simulink model "positionWalking_legacy"  (Simulink 8.3)
settings: Solver=FixedStepDiscrete  StartTime=0.0  StopTime=Config.t_end  FixedStep=Config.t_step  RelTol=1e-3
InitFcn:
  | cd(fileparts(which(bdroot)));
  | initTorqueWalking;
undefined symbols (not defined in the file): Config, DiscIntNeverNeededParam, gains, ROBOT_DOF
libraries: WBToolboxLibrary x88
(part 2 of 3)

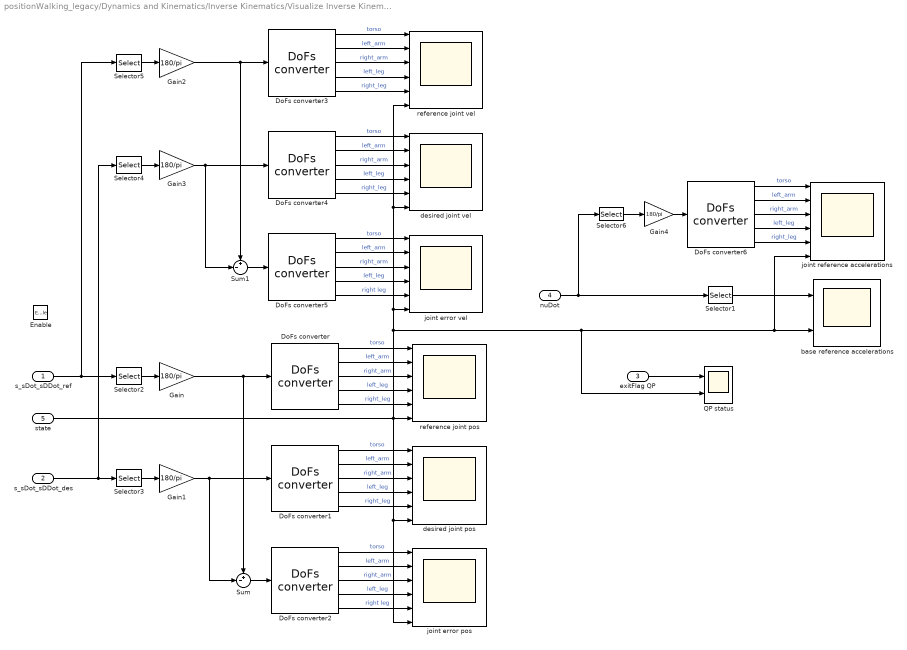
== system positionWalking_legacy/Dynamics and Kinematics/Inverse Kinematics/Visualize Inverse Kinematics ==
  s_sDot_sDDot_ref : Inport
  s_sDot_sDDot_des : Inport  Port=2
  exitFlag QP : Inport  Port=3
  nuDot : Inport  Port=4
  state : Inport  Port=5
  Enable : EnablePort
  DoFs converter{,1..6} (7 alike) : WBToolboxLibrary/Utilities/DoFs converter  yarp2WBIOption=From WBI to YARP  robotName=WBT_robotName  localName=WBT_modelName  wbiFile=WBT_wbiFilename  wbiList=WBT_wbiList
  Gain{,1..4} (5 alike) : Gain  Gain=180/pi
  QP status : Scope  NumInputPorts=2
      settings: TimeRange=auto  MaxDataPoints=5000  SaveName=ikin_QPStatus_DATA  YMin=-1.00000~0.9  YMax=1.00000~1.1  SampleTime=-1
  Selector1 : Selector  InputPortWidth=ROBOT_DOF+6  IndexOptions=Index vector (dialog)  Indices=[1:6]  OutputSizes=1
  Selector2 : Selector  NumberOfDimensions=2  InputPortWidth=ROBOT_DOF  IndexOptions=Index vector (dialog),Index vector (dialog)  Indices=[1:ROBOT_DOF],1  OutputSizes=1,1
  Selector3 : Selector  NumberOfDimensions=2  InputPortWidth=ROBOT_DOF  IndexOptions=Index vector (dialog),Index vector (dialog)  Indices=[1:ROBOT_DOF],1  OutputSizes=1,1
  Selector4 : Selector  NumberOfDimensions=2  InputPortWidth=ROBOT_DOF  IndexOptions=Index vector (dialog),Index vector (dialog)  Indices=[1:ROBOT_DOF],2  OutputSizes=1,1
  Selector5 : Selector  NumberOfDimensions=2  InputPortWidth=ROBOT_DOF  IndexOptions=Index vector (dialog),Index vector (dialog)  Indices=[1:ROBOT_DOF],2  OutputSizes=1,1
  Selector6 : Selector  InputPortWidth=ROBOT_DOF+6  IndexOptions=Index vector (dialog)  Indices=[7:ROBOT_DOF+6]  OutputSizes=1
  Sum : Sum  Inputs=+-|
  Sum1 : Sum  Inputs=+-|
  base reference accelerations : Scope  NumInputPorts=2
      settings: TimeRange=auto  MaxDataPoints=5000  SaveName=ikin_baseAcc_DATA  YMin=-0.01102~0.9  YMax=0.00514~1.1  SampleTime=-1
  desired joint pos : Scope  NumInputPorts=6
      settings: TimeRange=auto  ShowLegends=on  MaxDataPoints=5000  SaveName=ikin_s_des_DATA  YMin=-0.00195~-39.1214~-39.1221~-0.14128~-0.12031~0.9  YMax=0.02043~54.3146~54.31552~0.12783~0.13205~1.1  SampleTime=-1
  desired joint vel : Scope  NumInputPorts=6
      settings: TimeRange=auto  MaxDataPoints=5000  SaveName=ikin_sDot_des_DATA  YMin=-1.00000~-1.00000~-1.00000~-1.00000~-1.00000~0.9  YMax=1.00000~1.00000~1.00000~1.00000~1.00000~1.1  SampleTime=-1
  joint error pos : Scope  NumInputPorts=6
      settings: TimeRange=auto  MaxDataPoints=5000  SaveName=ikin_s_err_DATA  YMin=-5.9022~-0.98644~-1.02648~-5.57984~-5.5405~0.9  YMax=6.12835~0.97735~0.94334~5.54057~5.57971~1.1  SampleTime=-1
  joint error vel : Scope  NumInputPorts=6
      settings: TimeRange=auto  MaxDataPoints=5000  SaveName=ikin_sDot_err_DATA  YMin=-0.00011~-0.000021~-0.00064~-0.00028~-0.00066~0.9  YMax=0.00008~0.000046~0.00101~0.00072~0.00021~1.1  SampleTime=-1
  joint reference accelerations : Scope  NumInputPorts=6
      settings: TimeRange=auto  MaxDataPoints=5000  SaveName=ikin_sDDot_ref_DATA  YMin=-2.86444~-1.31048~-1.31054~-1.0443~-1.04238~0.9  YMax=1.2637~1.01756~1.0173~0.54022~0.54065~1.1  SampleTime=-1
  reference joint pos : Scope  NumInputPorts=6
      settings: TimeRange=auto  MaxDataPoints=5000  SaveName=ikin_s_ref_DATA  YMin=-1.73238~-39.09396~-39.16347~-0.13035~-0.1588~0.9  YMax=-0.13168~54.24597~54.26229~0.09217~0.03558~1.1  SampleTime=-1
  reference joint vel : Scope  NumInputPorts=6
      settings: TimeRange=auto  MaxDataPoints=5000  SaveName=ikin_sDot_ref_DATA  YMin=-1.00000~-1.00000~-1.00000~-1.00000~-1.00000~0.9  YMax=1.00000~1.00000~1.00000~1.00000~1.00000~1.1  SampleTime=-1
  wires:
  DoFs converter1/2 -> desired joint pos/2  "left_arm"
  DoFs converter/5 -> reference joint pos/5  "right_leg"
  DoFs converter2/1 -> joint error pos/1  "torso"
  DoFs converter/4 -> reference joint pos/4  "left_leg"
  DoFs converter/2 -> reference joint pos/2  "left_arm"
  DoFs converter1/1 -> desired joint pos/1  "torso"
  DoFs converter1/4 -> desired joint pos/4  "left_leg"
  DoFs converter1/3 -> desired joint pos/3  "right_arm"
  DoFs converter/3 -> reference joint pos/3  "right_arm"
  DoFs converter2/2 -> joint error pos/2  "left_arm"
  DoFs converter/1 -> reference joint pos/1  "torso"
  DoFs converter1/5 -> desired joint pos/5  "right_leg"
  DoFs converter2/4 -> joint error pos/4  "left_leg"
  Sum/1 -> DoFs converter2/1
  DoFs converter2/3 -> joint error pos/3  "right_arm"
  Gain/1 -> Sum/1, DoFs converter/1
  Gain1/1 -> Sum/2, DoFs converter1/1
  DoFs converter4/2 -> desired joint vel/2  "left_arm"
  DoFs converter3/5 -> reference joint vel/5  "right_leg"
  DoFs converter5/1 -> joint error vel/1  "torso"
  DoFs converter3/4 -> reference joint vel/4  "left_leg"
  DoFs converter3/2 -> reference joint vel/2  "left_arm"
  s_sDot_sDDot_ref/1 -> Selector5/1, Selector2/1
  DoFs converter4/1 -> desired joint vel/1  "torso"
  DoFs converter4/4 -> desired joint vel/4  "left_leg"
  DoFs converter4/3 -> desired joint vel/3  "right_arm"
  DoFs converter3/3 -> reference joint vel/3  "right_arm"
  DoFs converter5/2 -> joint error vel/2  "left_arm"
  DoFs converter3/1 -> reference joint vel/1  "torso"
  s_sDot_sDDot_des/1 -> Selector4/1, Selector3/1
  DoFs converter4/5 -> desired joint vel/5  "right_leg"
  DoFs converter5/4 -> joint error vel/4  "left_leg"
  Sum1/1 -> DoFs converter5/1
  DoFs converter5/3 -> joint error vel/3  "right_arm"
  Gain2/1 -> Sum1/1, DoFs converter3/1
  Gain3/1 -> Sum1/2, DoFs converter4/1
  DoFs converter5/5 -> joint error vel/5  "right leg"
  DoFs converter2/5 -> joint error pos/5  "right leg"
  Selector1/1 -> base reference accelerations/1
  Selector2/1 -> Gain/1
  Selector3/1 -> Gain1/1
  Selector4/1 -> Gain3/1
  Selector5/1 -> Gain2/1
  DoFs converter6/5 -> joint reference accelerations/5  "right_leg"
  DoFs converter6/1 -> joint reference accelerations/1  "torso"
  DoFs converter6/4 -> joint reference accelerations/4  "left_leg"
  DoFs converter6/3 -> joint reference accelerations/3  "right_arm"
  DoFs converter6/2 -> joint reference accelerations/2  "left_arm"
  nuDot/1 -> Selector6/1, Selector1/1
  Gain4/1 -> DoFs converter6/1
  Selector6/1 -> Gain4/1
  state/1 -> reference joint vel/6, desired joint vel/6, joint error vel/6, QP status/2, joint reference accelerations/6, base reference accelerations/2, joint error pos/6, desired joint pos/6, reference joint pos/6
  exitFlag QP/1 -> QP status/1

== system positionWalking_legacy/Dynamics and Kinematics/Task Accelerations/ComputeTasksPoseAndVelocity ==
  J_LFoot : Inport
  J_RFoot : Inport  Port=2
  J_CoM : Inport  Port=3
  J_Rot_task : Inport  Port=4
  s : Inport  Port=5
  w_H_b : Inport  Port=6
  nu : Inport  Port=7
  Compose Task Pose and Velocity : MATLAB Function  TreatAsAtomicUnit=on
      settings: PermitHierarchicalResolution=ParametersOnly
  Product{,1..3} (4 alike) : Product  Multiplication=Matrix(*)
  Task position and orientation : Subsystem
  pos_vel_CoM : Outport
  pose_vel_LFoot : Outport  Port=2
  pose_vel_RFoot : Outport  Port=3
  orient_vel_Rot_task : Outport  Port=4
  wires:
  Compose Task Pose and Velocity/3(pose_vel_RFoot) -> pose_vel_RFoot/1
  Compose Task Pose and Velocity/2(pose_vel_LFoot) -> pose_vel_LFoot/1
  Compose Task Pose and Velocity/1(pos_vel_CoM) -> pos_vel_CoM/1
  Compose Task Pose and Velocity/4(orient_vel_Rot_task) -> orient_vel_Rot_task/1
  nu/1 -> Product1/2, Product/2, Product2/2, Product3/2
  J_Rot_task/1 -> Product3/1
  Product/1 -> Compose Task Pose and Velocity/1(vel_CoM)
  Product1/1 -> Compose Task Pose and Velocity/2(vel_LFoot)
  Product2/1 -> Compose Task Pose and Velocity/3(vel_RFoot)
  Product3/1 -> Compose Task Pose and Velocity/4(vel_Rot_task)
  s/1 -> Task position and orientation/1(s)
  w_H_b/1 -> Task position and orientation/2(w_H_b)
  Task position and orientation/1(w_H_CoM) -> Compose Task Pose and Velocity/5(w_H_CoM)
  Task position and orientation/2(w_H_l_sole) -> Compose Task Pose and Velocity/6(w_H_l_sole)
  Task position and orientation/3(w_H_r_sole) -> Compose Task Pose and Velocity/7(w_H_r_sole)
  Task position and orientation/4(w_H_Rot_task) -> Compose Task Pose and Velocity/8(w_H_Rot_task)
  J_RFoot/1 -> Product2/1
  J_LFoot/1 -> Product1/1
  J_CoM/1 -> Product/1

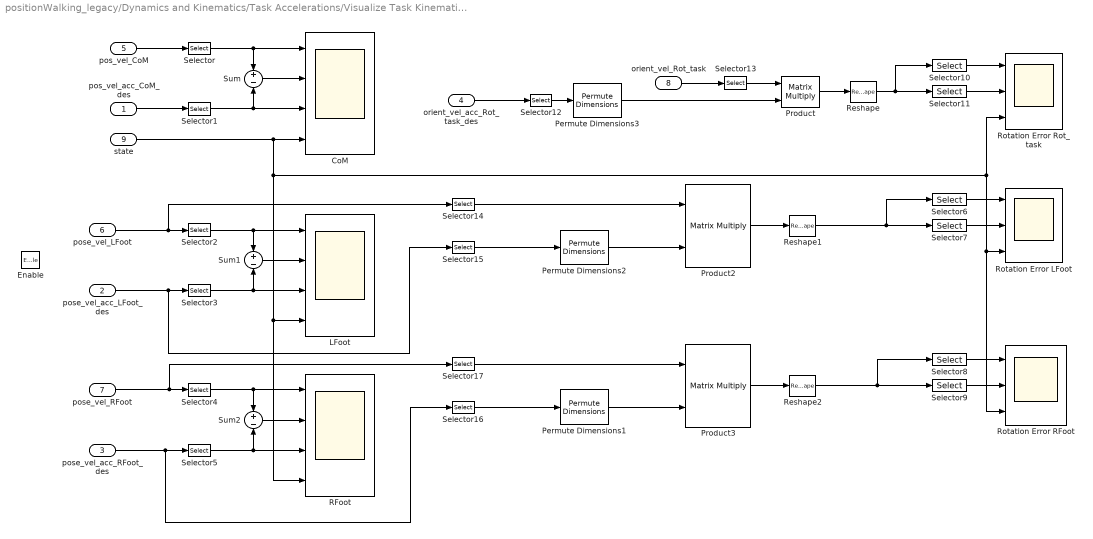
== system positionWalking_legacy/Dynamics and Kinematics/Task Accelerations/Visualize Task Kinematics ==
  pos_vel_acc_CoM_des : Inport
  pose_vel_acc_LFoot_des : Inport  Port=2
  pose_vel_acc_RFoot_des : Inport  Port=3
  orient_vel_acc_Rot_task_des : Inport  Port=4
  pos_vel_CoM : Inport  Port=5
  pose_vel_LFoot : Inport  Port=6
  pose_vel_RFoot : Inport  Port=7
  orient_vel_Rot_task : Inport  Port=8
  state : Inport  Port=9
  Enable : EnablePort
  CoM : Scope  NumInputPorts=4
      settings: TimeRange=auto  MaxDataPoints=5000  SaveName=forKin_CoM_DATA  YMin=-0.16396~-0.00327~-0.16319~0.9  YMax=0.58824~0.00906~0.58815~1.1  SampleTime=-1
  LFoot : Scope  NumInputPorts=4
      settings: TimeRange=auto  MaxDataPoints=5000  SaveName=forKin_LFoot_DATA  YMin=-0.00000000000000042~-0.00000000000000042~-0.000000000000000002~0.9  YMax=0.00000000000000045~0.00000000000000045~0.000000000000000017~1.1  SampleTime=-1
  Permute Dimensions1 : PermuteDimensions
  Permute Dimensions2 : PermuteDimensions
  Permute Dimensions3 : PermuteDimensions
  Product : Product  Multiplication=Matrix(*)
  Product2 : Product  Multiplication=Matrix(*)
  Product3 : Product  Multiplication=Matrix(*)
  RFoot : Scope  NumInputPorts=4
      settings: TimeRange=auto  MaxDataPoints=5000  SaveName=forKin_RFoot_DATA  YMin=-0.15347~-0.00033~-0.15317~0.9  YMax=0.01708~0.00035~0.01701~1.1  SampleTime=-1
  Reshape : Reshape
  Reshape1 : Reshape
  Reshape2 : Reshape
  Rotation Error LFoot : Scope  NumInputPorts=3
      settings: TimeRange=auto  MaxDataPoints=5000  SaveName=rotErr_LFoot_DATA  YMin=0.9999999999999994~-0.00000000000000006~0.9  YMax=1.0000000000000009~0.00000000000000006~1.1  SampleTime=-1
  Rotation Error RFoot : Scope  NumInputPorts=3
      settings: TimeRange=auto  MaxDataPoints=5000  SaveName=rotErr_RFoot_DATA  YMin=0.99999975~-0.00082~0.9  YMax=1.00000003~0.00082~1.1  SampleTime=-1
  Rotation Error Rot_task : Scope  NumInputPorts=3
      settings: TimeRange=auto  MaxDataPoints=5000  SaveName=rotErr_Root_DATA  YMin=0.99623~-0.1023~0.9  YMax=1.00042~0.1023~1.1  SampleTime=-1
  Selector{,1..5} (6 alike) : Selector  NumberOfDimensions=2  InputPortWidth=3  IndexOptions=Index vector (dialog),Index vector (dialog)  Indices=[1:3],1  OutputSizes=1,1
  Selector10 : Selector  InputPortWidth=9  IndexOptions=Index vector (dialog)  Indices=[1 5 9]  OutputSizes=1
  Selector11 : Selector  InputPortWidth=9  IndexOptions=Index vector (dialog)  Indices=[2 3 4 6 7 8]  OutputSizes=1
  Selector12 : Selector  NumberOfDimensions=2  InputPortWidth=3  IndexOptions=Index vector (dialog),Index vector (dialog)  Indices=[1:3],[1:3]  OutputSizes=1,1
  Selector13 : Selector  NumberOfDimensions=2  InputPortWidth=3  IndexOptions=Index vector (dialog),Index vector (dialog)  Indices=[1:3],[1:3]  OutputSizes=1,1
  Selector{14..17} (4 alike) : Selector  NumberOfDimensions=2  InputPortWidth=3  IndexOptions=Index vector (dialog),Index vector (dialog)  Indices=[4:6],[1:3]  OutputSizes=1,1
  Selector6 : Selector  InputPortWidth=9  IndexOptions=Index vector (dialog)  Indices=[1 5 9]  OutputSizes=1
  Selector7 : Selector  InputPortWidth=9  IndexOptions=Index vector (dialog)  Indices=[2 3 4 6 7 8]  OutputSizes=1
  Selector8 : Selector  InputPortWidth=9  IndexOptions=Index vector (dialog)  Indices=[1 5 9]  OutputSizes=1
  Selector9 : Selector  InputPortWidth=9  IndexOptions=Index vector (dialog)  Indices=[2 3 4 6 7 8]  OutputSizes=1
  Sum : Sum  Inputs=+|-
  Sum1 : Sum  Inputs=+|-
  Sum2 : Sum  Inputs=+|-
  wires:
  Selector/1 -> Sum/1, CoM/1
  Selector1/1 -> CoM/3, Sum/2
  Sum/1 -> CoM/2
  pos_vel_CoM/1 -> Selector/1
  pos_vel_acc_CoM_des/1 -> Selector1/1
  Selector2/1 -> LFoot/1, Sum1/1
  Selector3/1 -> LFoot/3, Sum1/2
  Sum1/1 -> LFoot/2
  Selector4/1 -> RFoot/1, Sum2/1
  Selector5/1 -> RFoot/3, Sum2/2
  Sum2/1 -> RFoot/2
  pose_vel_RFoot/1 -> Selector17/1, Selector4/1
  state/1 -> RFoot/4, LFoot/4, Rotation Error RFoot/3, Rotation Error LFoot/3, Rotation Error Rot_task/3, CoM/4
  pose_vel_acc_RFoot_des/1 -> Selector5/1, Selector16/1
  Permute Dimensions2/1 -> Product2/2
  Permute Dimensions1/1 -> Product3/2
  Permute Dimensions3/1 -> Product/2
  Product2/1 -> Reshape1/1
  Product3/1 -> Reshape2/1
  Product/1 -> Reshape/1
  Selector13/1 -> Product/1
  pose_vel_LFoot/1 -> Selector14/1, Selector2/1
  Reshape1/1 -> Selector6/1, Selector7/1
  Reshape2/1 -> Selector8/1, Selector9/1
  Reshape/1 -> Selector10/1, Selector11/1
  Selector7/1 -> Rotation Error LFoot/2
  Selector6/1 -> Rotation Error LFoot/1
  Selector8/1 -> Rotation Error RFoot/1
  Selector9/1 -> Rotation Error RFoot/2
  Selector10/1 -> Rotation Error Rot_task/1
  Selector11/1 -> Rotation Error Rot_task/2
  Selector12/1 -> Permute Dimensions3/1
  pose_vel_acc_LFoot_des/1 -> Selector15/1, Selector3/1
  orient_vel_acc_Rot_task_des/1 -> Selector12/1
  orient_vel_Rot_task/1 -> Selector13/1
  Selector14/1 -> Product2/1
  Selector15/1 -> Permute Dimensions2/1
  Selector16/1 -> Permute Dimensions1/1
  Selector17/1 -> Product3/1

== system positionWalking_legacy/Robot State and References/Reference Velocities and Accelerations/Reference Orientations ==
  w_R_LFoot_des : Inport
  w_R_RFoot_des : Inport  Port=2
  w_R_Rot_task_des : Inport  Port=3
  Compute Reference Angular Accelerations : MATLAB Function  TreatAsAtomicUnit=on
      settings: PermitHierarchicalResolution=ParametersOnly
  Compute Rotation Matrix Derivative : MATLAB Function  TreatAsAtomicUnit=on
      settings: PermitHierarchicalResolution=ParametersOnly
  Discrete-Time Integrator : DiscreteIntegrator  InitialCondition=zeros(3,1)  InitialConditionSetting=State (most efficient)  SampleTime=Config.t_step  ICPrevOutput=DiscIntNeverNeededParam  ICPrevScaledInput=DiscIntNeverNeededParam
  Discrete-Time Integrator1 : DiscreteIntegrator  InitialConditionSource=external  InitialCondition=zeros(3,1)  InitialConditionSetting=State (most efficient)  SampleTime=Config.t_step  ICPrevOutput=DiscIntNeverNeededParam  ICPrevScaledInput=DiscIntNeverNeededParam
  Discrete-Time Integrator2 : DiscreteIntegrator  InitialConditionSource=external  InitialCondition=zeros(3,1)  InitialConditionSetting=State (most efficient)  SampleTime=Config.t_step  ICPrevOutput=DiscIntNeverNeededParam  ICPrevScaledInput=DiscIntNeverNeededParam
  Discrete-Time Integrator3 : DiscreteIntegrator  InitialCondition=zeros(3,1)  InitialConditionSetting=State (most efficient)  SampleTime=Config.t_step  ICPrevOutput=DiscIntNeverNeededParam  ICPrevScaledInput=DiscIntNeverNeededParam
  Discrete-Time Integrator4 : DiscreteIntegrator  InitialCondition=zeros(3,1)  InitialConditionSetting=State (most efficient)  SampleTime=Config.t_step  ICPrevOutput=DiscIntNeverNeededParam  ICPrevScaledInput=DiscIntNeverNeededParam
  Discrete-Time Integrator5 : DiscreteIntegrator  InitialConditionSource=external  InitialCondition=zeros(3,1)  InitialConditionSetting=State (most efficient)  SampleTime=Config.t_step  ICPrevOutput=DiscIntNeverNeededParam  ICPrevScaledInput=DiscIntNeverNeededParam
  Matrix Concatenate5 : Concatenate  NumInputs=3  Mode=Multidimensional array  ConcatenateDimension=2
  Matrix Concatenate6 : Concatenate  NumInputs=3  Mode=Multidimensional array  ConcatenateDimension=2
  Matrix Concatenate7 : Concatenate  NumInputs=3  Mode=Multidimensional array  ConcatenateDimension=2
  Visualize Desired Rotations : Subsystem
  "holder " : WBToolboxLibrary/Utilities/holder 
  holder 1 : WBToolboxLibrary/Utilities/holder 
  holder 2 : WBToolboxLibrary/Utilities/holder 
  orient_vel_acc_LFoot_des : Outport
  orient_vel_acc_RFoot_des : Outport  Port=2
  orient_vel_acc_Rot_task_des : Outport  Port=3
  wires:
  Compute Reference Angular Accelerations/1(omegaDot_LFoot) -> Discrete-Time Integrator/1, Matrix Concatenate6/3, Visualize Desired Rotations/4(omegaDot_LFoot)
  Compute Reference Angular Accelerations/3(omegaDot_Rot_task) -> Discrete-Time Integrator4/1, Matrix Concatenate7/3, Visualize Desired Rotations/6(omegaDot_Root)
  Discrete-Time Integrator/1 -> Compute Rotation Matrix Derivative/1(omega_LFoot), Matrix Concatenate6/2, Compute Reference Angular Accelerations/7(omega_LFoot), Visualize Desired Rotations/9(omega_LFoot)
  Discrete-Time Integrator3/1 -> Compute Rotation Matrix Derivative/2(omega_RFoot), Matrix Concatenate5/2, Compute Reference Angular Accelerations/8(omega_RFoot), Visualize Desired Rotations/8(omega_RFoot)
  Discrete-Time Integrator4/1 -> Compute Rotation Matrix Derivative/3(omega_Rot_task), Matrix Concatenate7/2, Compute Reference Angular Accelerations/9(omega_Rot_task), Visualize Desired Rotations/7(omega_Rot_task)
  Compute Rotation Matrix Derivative/1(RDot_LFoot) -> Discrete-Time Integrator2/1
  Compute Rotation Matrix Derivative/2(RDot_RFoot) -> Discrete-Time Integrator5/1
  Compute Rotation Matrix Derivative/3(RDot_Rot_task) -> Discrete-Time Integrator1/1
  Discrete-Time Integrator2/1 -> Compute Rotation Matrix Derivative/4(w_R_LFoot), Matrix Concatenate6/1, Visualize Desired Rotations/10(w_R_LFoot), Compute Reference Angular Accelerations/4(w_R_LFoot)
  Discrete-Time Integrator5/1 -> Compute Rotation Matrix Derivative/5(w_R_RFoot), Compute Reference Angular Accelerations/5(w_R_RFoot), Visualize Desired Rotations/11(w_R_RFoot), Matrix Concatenate5/1
  Discrete-Time Integrator1/1 -> Compute Rotation Matrix Derivative/6(w_R_Rot_task), Compute Reference Angular Accelerations/6(w_R_Rot_task), Matrix Concatenate7/1, Visualize Desired Rotations/12(w_R_Rot_task)
  "holder "/1 -> Discrete-Time Integrator2/2
  holder 2/1 -> Discrete-Time Integrator5/2
  holder 1/1 -> Discrete-Time Integrator1/2
  Compute Reference Angular Accelerations/2(omegaDot_RFoot) -> Discrete-Time Integrator3/1, Matrix Concatenate5/3, Visualize Desired Rotations/5(omegaDot_RFoot)
  Matrix Concatenate6/1 -> orient_vel_acc_LFoot_des/1
  Matrix Concatenate5/1 -> orient_vel_acc_RFoot_des/1
  Matrix Concatenate7/1 -> orient_vel_acc_Rot_task_des/1
  w_R_LFoot_des/1 -> Visualize Desired Rotations/1(w_R_LFoot_des), "holder "/1, Compute Reference Angular Accelerations/1(w_R_LFoot_des)
  w_R_RFoot_des/1 -> Compute Reference Angular Accelerations/2(w_R_RFoot_des), Visualize Desired Rotations/2(w_R_RFoot_des), holder 2/1
  w_R_Rot_task_des/1 -> Compute Reference Angular Accelerations/3(w_R_Rot_task_des), Visualize Desired Rotations/3(w_R_Rot_task_des), holder 1/1

== system positionWalking_legacy/Robot State and References/Reference Velocities and Accelerations/Reference Positions ==
  pos_CoM_des : Inport
  pos_LFoot_des : Inport  Port=2
  pos_RFoot_des : Inport  Port=3
  s_des : Inport  Port=4
  Matrix Concatenate1 : Concatenate  NumInputs=3  Mode=Multidimensional array  ConcatenateDimension=2
  Matrix Concatenate2 : Concatenate  NumInputs=4  Mode=Multidimensional array  ConcatenateDimension=2
  Matrix Concatenate3 : Concatenate  NumInputs=4  Mode=Multidimensional array  ConcatenateDimension=2
  Matrix Concatenate4 : Concatenate  NumInputs=3  Mode=Multidimensional array  ConcatenateDimension=2
  Minimum Jerk Trajectory Generator{,1..3} (4 alike) : WBToolboxLibrary/Utilities/Minimum Jerk Trajectory Generator  externalSettlingTime=on  settlingTime=3  sampleTime=Config.t_step  resetOnSettlingTime=off  firstDerivatives=on  secondDerivatives=on  explicitInitialValue=off
  Settling time1 : Constant  Value=zeros(3,2)
  gains smoothing time : Constant  Value=Config.t_smoothingTimeRef
  pos_vel_acc_CoM_des : Outport
  s_sDot_sDDot_ref : Outport  Port=2
  pos_vel_acc_LFoot_des : Outport  Port=3
  pos_vel_acc_RFoot_des : Outport  Port=4
  wires:
  Minimum Jerk Trajectory Generator2/2 -> Matrix Concatenate3/2
  pos_LFoot_des/1 -> Minimum Jerk Trajectory Generator2/1
  pos_RFoot_des/1 -> Minimum Jerk Trajectory Generator3/1
  Minimum Jerk Trajectory Generator2/3 -> Matrix Concatenate3/3
  Minimum Jerk Trajectory Generator2/1 -> Matrix Concatenate3/1
  Minimum Jerk Trajectory Generator1/3 -> Matrix Concatenate1/3
  Matrix Concatenate1/1 -> s_sDot_sDDot_ref/1
  Matrix Concatenate4/1 -> pos_vel_acc_CoM_des/1
  Minimum Jerk Trajectory Generator1/1 -> Matrix Concatenate1/1
  pos_CoM_des/1 -> Minimum Jerk Trajectory Generator/1
  Minimum Jerk Trajectory Generator/3 -> Matrix Concatenate4/3
  Minimum Jerk Trajectory Generator/2 -> Matrix Concatenate4/2
  Minimum Jerk Trajectory Generator1/2 -> Matrix Concatenate1/2
  Minimum Jerk Trajectory Generator3/3 -> Matrix Concatenate2/3
  Matrix Concatenate3/1 -> pos_vel_acc_LFoot_des/1
  Matrix Concatenate2/1 -> pos_vel_acc_RFoot_des/1
  Minimum Jerk Trajectory Generator/1 -> Matrix Concatenate4/1
  Minimum Jerk Trajectory Generator3/2 -> Matrix Concatenate2/2
  s_des/1 -> Minimum Jerk Trajectory Generator1/1
  Settling time1/1 -> Matrix Concatenate2/4, Matrix Concatenate3/4
  gains smoothing time/1 -> Minimum Jerk Trajectory Generator/2, Minimum Jerk Trajectory Generator1/2, Minimum Jerk Trajectory Generator2/2, Minimum Jerk Trajectory Generator3/2
  Minimum Jerk Trajectory Generator3/1 -> Matrix Concatenate2/1

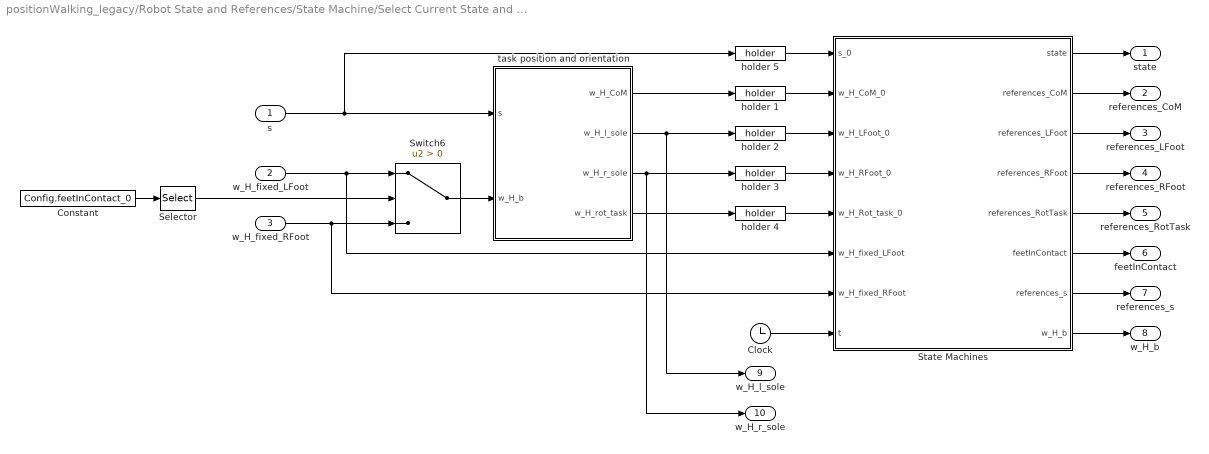
== system positionWalking_legacy/Robot State and References/State Machine/Select Current State and References ==
  s : Inport
  w_H_fixed_LFoot : Inport  Port=2
  w_H_fixed_RFoot : Inport  Port=3
  Clock : Clock
  Constant : Constant  Value=Config.feetInContact_0
  Selector : Selector  InputPortWidth=2  IndexOptions=Index vector (dialog)  Indices=1  OutputSizes=1
  State Machines : MATLAB Function  TreatAsAtomicUnit=on
      settings: PermitHierarchicalResolution=ParametersOnly
  Switch6 : Switch  Criteria=u2 > Threshold
  holder {1..5} (5 alike) : WBToolboxLibrary/Utilities/holder 
  task position and orientation : Subsystem
  state : Outport
  references_CoM : Outport  Port=2
  references_LFoot : Outport  Port=3
  references_RFoot : Outport  Port=4
  references_RotTask : Outport  Port=5
  feetInContact : Outport  Port=6
  references_s : Outport  Port=7
  w_H_b : Outport  Port=8
  w_H_l_sole : Outport  Port=9
  w_H_r_sole : Outport  Port=10
  wires:
  Switch6/1 -> task position and orientation/2(w_H_b)
  w_H_fixed_LFoot/1 -> Switch6/1, State Machines/6(w_H_fixed_LFoot)
  Constant/1 -> Selector/1
  State Machines/3(references_LFoot) -> references_LFoot/1
  task position and orientation/2(w_H_l_sole) -> holder 2/1, w_H_l_sole/1
  holder 3/1 -> State Machines/4(w_H_RFoot_0)
  State Machines/5(references_RotTask) -> references_RotTask/1
  State Machines/4(references_RFoot) -> references_RFoot/1
  s/1 -> task position and orientation/1(s), holder 5/1
  holder 4/1 -> State Machines/5(w_H_Rot_task_0)
  task position and orientation/1(w_H_CoM) -> holder 1/1
  holder 2/1 -> State Machines/3(w_H_LFoot_0)
  task position and orientation/4(w_H_rot_task) -> holder 4/1
  Selector/1 -> Switch6/2
  State Machines/1(state) -> state/1
  w_H_fixed_RFoot/1 -> State Machines/7(w_H_fixed_RFoot), Switch6/3
  State Machines/6(feetInContact) -> feetInContact/1
  task position and orientation/3(w_H_r_sole) -> holder 3/1, w_H_r_sole/1
  Clock/1 -> State Machines/8(t)
  State Machines/7(references_s) -> references_s/1
  State Machines/2(references_CoM) -> references_CoM/1
  State Machines/8(w_H_b) -> w_H_b/1
  holder 1/1 -> State Machines/2(w_H_CoM_0)
  holder 5/1 -> State Machines/1(s_0)

== system positionWalking_legacy/Robot State and References/State Machine/World to fixed link transform ==
  s : Inport
  w_H_b : Inport  Port=2
  IMU port : Inport  Port=3
  left foot : WBToolboxLibrary/wholeBodyModel/Kinematics/Forward Kinematics  frameName=Frames.LEFT_FOOT  robotName=WBT_robotName  localName=WBT_modelName  wbiFile=WBT_wbiFilename  wbiList=WBT_wbiList
  right foot : WBToolboxLibrary/wholeBodyModel/Kinematics/Forward Kinematics  frameName=Frames.RIGHT_FOOT  robotName=WBT_robotName  localName=WBT_modelName  wbiFile=WBT_wbiFilename  wbiList=WBT_wbiList
  w_H_b with left foot fixed : Subsystem
  w_H_b with right foot fixed : Subsystem
  w_H_fixed_LFoot : Outport
  w_H_fixed_RFoot : Outport  Port=2
  wires:
  s/1 -> right foot/2, w_H_b with right foot fixed/1(s), w_H_b with left foot fixed/1(s), left foot/2
  w_H_b/1 -> left foot/1, right foot/1
  w_H_b with right foot fixed/1(w_H_b) -> w_H_fixed_RFoot/1
  IMU port/1 -> w_H_b with left foot fixed/2(inertial), w_H_b with right foot fixed/2(inertial)
  right foot/1 -> w_H_b with right foot fixed/3(w_H_fixedLink)
  w_H_b with left foot fixed/1(w_H_b) -> w_H_fixed_LFoot/1
  left foot/1 -> w_H_b with left foot fixed/3(w_H_fixedLink)

== system positionWalking_legacy/Robot State and References/State Machine/compute state velocity ==
  s : Inport
  w_H_b : Inport  Port=2
  "feetInContact " : Inport  Port=3
  Compute Base Velocity : MATLAB Function  TreatAsAtomicUnit=on
      settings: PermitHierarchicalResolution=ParametersOnly
  Feet Jacobians : Subsystem
  Get Estimate : WBToolboxLibrary/wholeBodyStates/Get Estimate  estimateType=Joints Velocity  robotName=WBT_robotName  localName=WBT_modelName  wbiFile=WBT_wbiFilename  wbiList=WBT_wbiList
  Mux : Mux  Inputs=2
  nu : Outport
  wires:
  Get Estimate/1 -> Mux/2, Compute Base Velocity/4(sDot)
  Mux/1 -> nu/1
  "feetInContact "/1 -> Compute Base Velocity/3(feetInContact)
  Compute Base Velocity/1(nu_b) -> Mux/1
  s/1 -> Feet Jacobians/1(s)
  w_H_b/1 -> Feet Jacobians/2(w_H_b)
  Feet Jacobians/1(J_LFoot) -> Compute Base Velocity/1(J_LeftFoot)
  Feet Jacobians/2(J_RFoot) -> Compute Base Velocity/2(J_RightFoot)

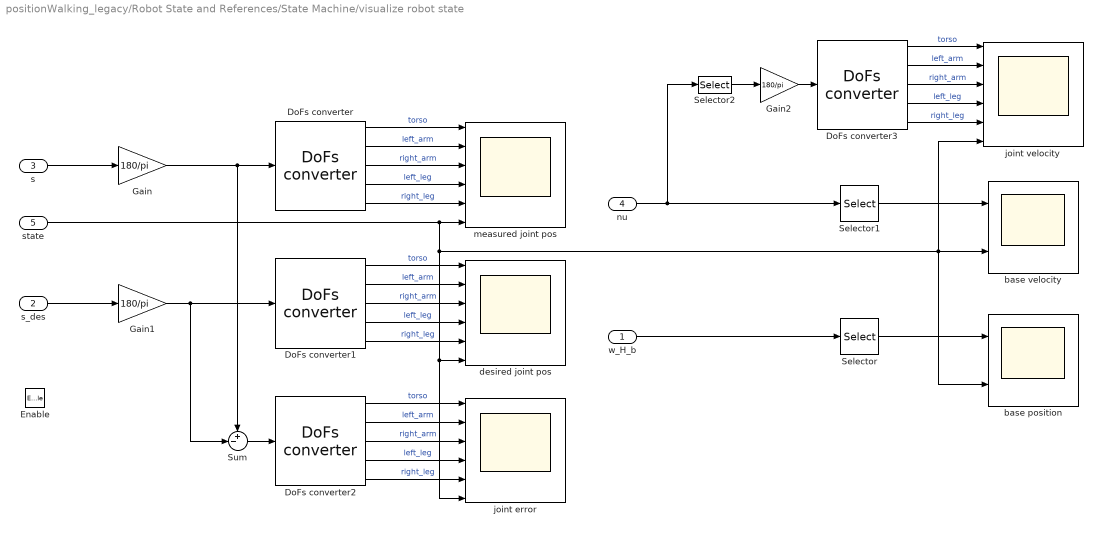
== system positionWalking_legacy/Robot State and References/State Machine/visualize robot state ==
  w_H_b : Inport
  s_des : Inport  Port=2
  s : Inport  Port=3
  nu : Inport  Port=4
  state : Inport  Port=5
  Enable : EnablePort
  DoFs converter{,1..3} (4 alike) : WBToolboxLibrary/Utilities/DoFs converter  yarp2WBIOption=From WBI to YARP  robotName=WBT_robotName  localName=WBT_modelName  wbiFile=WBT_wbiFilename  wbiList=WBT_wbiList
  Gain : Gain  Gain=180/pi
  Gain1 : Gain  Gain=180/pi
  Gain2 : Gain  Gain=180/pi
  Selector : Selector  NumberOfDimensions=2  InputPortWidth=3  IndexOptions=Index vector (dialog),Index vector (dialog)  Indices=[1:3],4  OutputSizes=1,1
  Selector1 : Selector  InputPortWidth=ROBOT_DOF+6  IndexOptions=Index vector (dialog)  Indices=[1:6]  OutputSizes=1
  Selector2 : Selector  InputPortWidth=ROBOT_DOF+6  IndexOptions=Index vector (dialog)  Indices=[7:ROBOT_DOF+6]  OutputSizes=1
  Sum : Sum  Inputs=+-|
  base position : Scope  NumInputPorts=2
      settings: TimeRange=auto  MaxDataPoints=5000  SaveName=basePos_DATA  YMin=-0.15075~0.9  YMax=0.68063~1.1  SampleTime=-1
  base velocity : Scope  NumInputPorts=2
      settings: TimeRange=auto  MaxDataPoints=5000  SaveName=baseVel_DATA  YMin=-0.00012~0.9  YMax=0.00016~1.1  SampleTime=-1
  desired joint pos : Scope  NumInputPorts=6
      settings: TimeRange=auto  MaxDataPoints=5000  SaveName=jointDes_DATA  YMin=-1.73238~-39.09396~-39.16347~-0.13035~-0.1588~0.9  YMax=-0.13168~54.24597~54.26229~0.09217~0.03558~1.1  SampleTime=-1
  joint error : Scope  NumInputPorts=6
      settings: TimeRange=auto  MaxDataPoints=5000  SaveName=jointErr_DATA  YMin=-0.10928~-0.03665~-0.06329~-0.00446~-0.00535~0.9  YMax=0.98348~0.04341~0.18869~0.01039~0.01469~1.1  SampleTime=-1
  joint velocity : Scope  NumInputPorts=6
      settings: TimeRange=auto  MaxDataPoints=5000  SaveName=jointVel_DATA  YMin=-0.03366~-0.02028~-0.03366~-0.01001~-0.00754~0.9  YMax=0.16882~0.03011~0.03479~0.00711~0.00828~1.1  SampleTime=-1
  measured joint pos : Scope  NumInputPorts=6
      settings: TimeRange=auto  MaxDataPoints=5000  SaveName=jointPos_DATA  YMin=-1.7483~-39.13033~-39.17068~-0.13107~-0.16256~0.9  YMax=0.01165~54.28691~54.29724~0.09225~0.036~1.1  SampleTime=-1
  wires:
  DoFs converter1/2 -> desired joint pos/2  "left_arm"
  DoFs converter/5 -> measured joint pos/5  "right_leg"
  DoFs converter2/1 -> joint error/1  "torso"
  DoFs converter/4 -> measured joint pos/4  "left_leg"
  DoFs converter/2 -> measured joint pos/2  "left_arm"
  s/1 -> Gain/1
  DoFs converter1/1 -> desired joint pos/1  "torso"
  DoFs converter1/4 -> desired joint pos/4  "left_leg"
  DoFs converter1/3 -> desired joint pos/3  "right_arm"
  DoFs converter/3 -> measured joint pos/3  "right_arm"
  DoFs converter2/5 -> joint error/5  "right_leg"
  DoFs converter2/2 -> joint error/2  "left_arm"
  DoFs converter/1 -> measured joint pos/1  "torso"
  s_des/1 -> Gain1/1
  DoFs converter1/5 -> desired joint pos/5  "right_leg"
  DoFs converter2/4 -> joint error/4  "left_leg"
  Sum/1 -> DoFs converter2/1
  DoFs converter2/3 -> joint error/3  "right_arm"
  DoFs converter3/5 -> joint velocity/5  "right_leg"
  DoFs converter3/1 -> joint velocity/1  "torso"
  DoFs converter3/4 -> joint velocity/4  "left_leg"
  DoFs converter3/3 -> joint velocity/3  "right_arm"
  DoFs converter3/2 -> joint velocity/2  "left_arm"
  nu/1 -> Selector2/1, Selector1/1
  w_H_b/1 -> Selector/1
  Gain/1 -> Sum/1, DoFs converter/1
  Gain1/1 -> Sum/2, DoFs converter1/1
  Gain2/1 -> DoFs converter3/1
  Selector/1 -> base position/1
  Selector2/1 -> Gain2/1
  state/1 -> measured joint pos/6, joint velocity/6, base velocity/2, base position/2, joint error/6, desired joint pos/6
  Selector1/1 -> base velocity/1

== system positionWalking_legacy/Dynamics and Kinematics/Initial Conditions/compute state velocity/Feet Jacobians ==
  s : Inport
  w_H_b : Inport  Port=2
  Jacobian LFoot : WBToolboxLibrary/wholeBodyModel/Jacobians/Jacobian  frameName=Frames.LEFT_FOOT  robotName=WBT_robotName  localName=WBT_modelName  wbiFile=WBT_wbiFilename  wbiList=WBT_wbiList
  Jacobian RFoot : WBToolboxLibrary/wholeBodyModel/Jacobians/Jacobian  frameName=Frames.RIGHT_FOOT  robotName=WBT_robotName  localName=WBT_modelName  wbiFile=WBT_wbiFilename  wbiList=WBT_wbiList
  J_LFoot : Outport
  J_RFoot : Outport  Port=2
  wires:
  Jacobian LFoot/1 -> J_LFoot/1
  Jacobian RFoot/1 -> J_RFoot/1
  w_H_b/1 -> Jacobian RFoot/1, Jacobian LFoot/1
  s/1 -> Jacobian LFoot/2, Jacobian RFoot/2

== system positionWalking_legacy/Dynamics and Kinematics/Inverse Kinematics/ComputeTasksPoseAndVelocity/Task position and orientation ==
  s : Inport
  w_H_b : Inport  Port=2
  CoM : WBToolboxLibrary/wholeBodyModel/Kinematics/Forward Kinematics  frameName=Frames.COM  robotName=WBT_robotName  localName=WBT_modelName  wbiFile=WBT_wbiFilename  wbiList=WBT_wbiList
  LFoot : WBToolboxLibrary/wholeBodyModel/Kinematics/Forward Kinematics  frameName=Frames.LEFT_FOOT  robotName=WBT_robotName  localName=WBT_modelName  wbiFile=WBT_wbiFilename  wbiList=WBT_wbiList
  RFoot : WBToolboxLibrary/wholeBodyModel/Kinematics/Forward Kinematics  frameName=Frames.RIGHT_FOOT  robotName=WBT_robotName  localName=WBT_modelName  wbiFile=WBT_wbiFilename  wbiList=WBT_wbiList
  Root : WBToolboxLibrary/wholeBodyModel/Kinematics/Forward Kinematics  frameName=Frames.ROT_TASK_LINK  robotName=WBT_robotName  localName=WBT_modelName  wbiFile=WBT_wbiFilename  wbiList=WBT_wbiList
  w_H_CoM : Outport
  w_H_l_sole : Outport  Port=2
  w_H_r_sole : Outport  Port=3
  w_H_Rot_task : Outport  Port=4
  wires:
  s/1 -> Root/2, RFoot/2, LFoot/2, CoM/2
  w_H_b/1 -> Root/1, CoM/1, LFoot/1, RFoot/1
  CoM/1 -> w_H_CoM/1
  LFoot/1 -> w_H_l_sole/1
  RFoot/1 -> w_H_r_sole/1
  Root/1 -> w_H_Rot_task/1

== system positionWalking_legacy/Dynamics and Kinematics/Inverse Kinematics/QP-Based Inverse Kinematics/QP Solver (inverse kinematics) ==
  Hessian : Inport
  gradient : Inport  Port=2
  ConstraintMatrix : Inport  Port=3
  biasVectorConstraint : Inport  Port=4
  QPSolver : M-S-Function  FunctionName=QPInverseKinematics  Parameters=ROBOT_DOF, Sat, Config
  nuDot : Outport
  ExitFlagQP : Outport  Port=2
  wires:
  QPSolver/1 -> nuDot/1
  QPSolver/2 -> ExitFlagQP/1
  Hessian/1 -> QPSolver/1
  gradient/1 -> QPSolver/2
  biasVectorConstraint/1 -> QPSolver/4
  ConstraintMatrix/1 -> QPSolver/3

== system positionWalking_legacy/Dynamics and Kinematics/Inverse Kinematics/QP-Based Inverse Kinematics/inverse kinematics integration ==
  nuDot : Inport
  nu_0 : Inport  Port=2
  q_0 : Inport  Port=3
  Compute Base Pose Derivative : MATLAB Function  TreatAsAtomicUnit=on
      settings: PermitHierarchicalResolution=ParametersOnly
  Demux : Demux  Outputs=[7;ROBOT_DOF]
  Demux1 : Demux  Outputs=[6; ROBOT_DOF]
  Integrate nu : DiscreteIntegrator  InitialConditionSource=external  SampleTime=Config.t_step  ICPrevOutput=DiscIntNeverNeededParam  ICPrevScaledInput=DiscIntNeverNeededParam
  Integrate nuDot : DiscreteIntegrator  InitialConditionSource=external  SampleTime=Config.t_step  ICPrevOutput=DiscIntNeverNeededParam  ICPrevScaledInput=DiscIntNeverNeededParam
  Matrix Concatenate : Concatenate  NumInputs=3  Mode=Multidimensional array  ConcatenateDimension=2
  Mux : Mux  Inputs=2
  Rewrite Base Pose as pos+quat : MATLAB Function  TreatAsAtomicUnit=on
      settings: PermitHierarchicalResolution=ParametersOnly
  Rewrite Base Pose as transformation matrix : MATLAB Function  TreatAsAtomicUnit=on
      settings: PermitHierarchicalResolution=ParametersOnly
  Selector3 : Selector  InputPortWidth=ROBOT_DOF+6  IndexOptions=Index vector (dialog)  Indices=[7:ROBOT_DOF+6]  OutputSizes=1
  Selector4 : Selector  InputPortWidth=ROBOT_DOF+6  IndexOptions=Index vector (dialog)  Indices=[7:ROBOT_DOF+6]  OutputSizes=1
  nu : Outport
  q : Outport  Port=2
  s_sDot_sDDot_des : Outport  Port=3
  wires:
  nu_0/1 -> Integrate nuDot/2
  q_0/1 -> Rewrite Base Pose as pos+quat/1(q_transf)
  nuDot/1 -> Selector4/1, Integrate nuDot/1
  Demux/1 -> Compute Base Pose Derivative/2(pose_b)
  Integrate nu/1 -> Demux/1, Rewrite Base Pose as transformation matrix/1(q_quat)
  Demux1/1 -> Compute Base Pose Derivative/1(nu_b)
  Compute Base Pose Derivative/1(pose_bDot) -> Mux/1
  Demux1/2 -> Mux/2
  Matrix Concatenate/1 -> s_sDot_sDDot_des/1
  Rewrite Base Pose as transformation matrix/1(q_transf) -> q/1
  Rewrite Base Pose as pos+quat/1(q_quat) -> Integrate nu/2
  Selector3/1 -> Matrix Concatenate/2
  Selector4/1 -> Matrix Concatenate/3
  Demux/2 -> Matrix Concatenate/1
  Mux/1 -> Integrate nu/1
  Integrate nuDot/1 -> Demux1/1, Selector3/1, nu/1

== system positionWalking_legacy/Dynamics and Kinematics/Task Accelerations/ComputeTasksPoseAndVelocity/Task position and orientation ==
  s : Inport
  w_H_b : Inport  Port=2
  CoM : WBToolboxLibrary/wholeBodyModel/Kinematics/Forward Kinematics  frameName=Frames.COM  robotName=WBT_robotName  localName=WBT_modelName  wbiFile=WBT_wbiFilename  wbiList=WBT_wbiList
  LFoot : WBToolboxLibrary/wholeBodyModel/Kinematics/Forward Kinematics  frameName=Frames.LEFT_FOOT  robotName=WBT_robotName  localName=WBT_modelName  wbiFile=WBT_wbiFilename  wbiList=WBT_wbiList
  RFoot : WBToolboxLibrary/wholeBodyModel/Kinematics/Forward Kinematics  frameName=Frames.RIGHT_FOOT  robotName=WBT_robotName  localName=WBT_modelName  wbiFile=WBT_wbiFilename  wbiList=WBT_wbiList
  Root : WBToolboxLibrary/wholeBodyModel/Kinematics/Forward Kinematics  frameName=Frames.ROT_TASK_LINK  robotName=WBT_robotName  localName=WBT_modelName  wbiFile=WBT_wbiFilename  wbiList=WBT_wbiList
  w_H_CoM : Outport
  w_H_l_sole : Outport  Port=2
  w_H_r_sole : Outport  Port=3
  w_H_Rot_task : Outport  Port=4
  wires:
  s/1 -> Root/2, RFoot/2, LFoot/2, CoM/2
  w_H_b/1 -> Root/1, CoM/1, LFoot/1, RFoot/1
  CoM/1 -> w_H_CoM/1
  LFoot/1 -> w_H_l_sole/1
  RFoot/1 -> w_H_r_sole/1
  Root/1 -> w_H_Rot_task/1

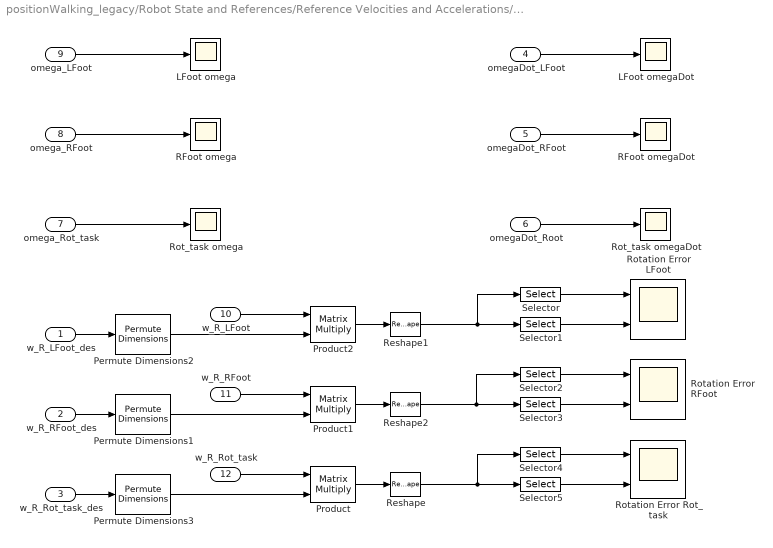
== system positionWalking_legacy/Robot State and References/Reference Velocities and Accelerations/Reference Orientations/Visualize Desired Rotations ==
  w_R_LFoot_des : Inport
  w_R_RFoot_des : Inport  Port=2
  w_R_Rot_task_des : Inport  Port=3
  omegaDot_LFoot : Inport  Port=4
  omegaDot_RFoot : Inport  Port=5
  omegaDot_Root : Inport  Port=6
  omega_Rot_task : Inport  Port=7
  omega_RFoot : Inport  Port=8
  omega_LFoot : Inport  Port=9
  w_R_LFoot : Inport  Port=10
  w_R_RFoot : Inport  Port=11
  w_R_Rot_task : Inport  Port=12
  LFoot omega : Scope
      settings: TimeRange=auto  MaxDataPoints=5000  SaveName=omega_LFoot_DATA  YMin=-0.000000000000000000000000000000000007  YMax=0.0000000000000000000000000000000000024  SampleTime=-1
  LFoot omegaDot : Scope
      settings: TimeRange=auto  MaxDataPoints=5000  SaveName=omegaDot_LFoot_DATA  YMin=-0.000000000000000000000000000000000014  YMax=0.000000000000000000000000000000000005  SampleTime=-1
  Permute Dimensions1 : PermuteDimensions
  Permute Dimensions2 : PermuteDimensions
  Permute Dimensions3 : PermuteDimensions
  Product : Product  Multiplication=Matrix(*)
  Product1 : Product  Multiplication=Matrix(*)
  Product2 : Product  Multiplication=Matrix(*)
  RFoot omega : Scope
      settings: TimeRange=auto  MaxDataPoints=5000  SaveName=omega_RFoot_DATA  YMin=-0.00000000000000000000003  YMax=0.00000000000000000000018  SampleTime=-1
  RFoot omegaDot : Scope
      settings: TimeRange=auto  MaxDataPoints=5000  SaveName=omegaDot_RFoot_DATA  YMin=-0.00000000000000000000015  YMax=0.00000000000000000000028  SampleTime=-1
  Reshape : Reshape
  Reshape1 : Reshape
  Reshape2 : Reshape
  Rot_task omega : Scope
      settings: TimeRange=auto  MaxDataPoints=5000  SaveName=omega_Root_DATA  YMin=-1.00000  YMax=1.00000  SampleTime=-1
  Rot_task omegaDot : Scope
      settings: TimeRange=auto  MaxDataPoints=5000  SaveName=omegaDot_Root_DATA  YMin=-1.00000  YMax=1.00000  SampleTime=-1
  Rotation Error LFoot : Scope  NumInputPorts=2
      settings: TimeRange=auto  MaxDataPoints=5000  SaveName=rotErr_LFoot_ref_DATA  YMin=0.9~-0.000000000000000000004  YMax=1.1~0.00000000000000000002  SampleTime=-1
  Rotation Error RFoot : Scope  NumInputPorts=2
      settings: TimeRange=auto  MaxDataPoints=5000  SaveName=rotError_RFoot_ref_DATA  YMin=0.9~-0.000000000000000069  YMax=2.00000~0.000000000000000008  SampleTime=-1
  Rotation Error Rot_task : Scope  NumInputPorts=2
      settings: TimeRange=auto  MaxDataPoints=5000  SaveName=rotErr_Root_ref_DATA  YMin=0.9~-0.0000000000000000024  YMax=1.1~0.0000000000000000041  SampleTime=-1
  Selector : Selector  InputPortWidth=9  IndexOptions=Index vector (dialog)  Indices=[1 5 9]  OutputSizes=1
  Selector1 : Selector  InputPortWidth=9  IndexOptions=Index vector (dialog)  Indices=[2 3 4 6 7 8]  OutputSizes=1
  Selector2 : Selector  InputPortWidth=9  IndexOptions=Index vector (dialog)  Indices=[1 5 9]  OutputSizes=1
  Selector3 : Selector  InputPortWidth=9  IndexOptions=Index vector (dialog)  Indices=[2 3 4 6 7 8]  OutputSizes=1
  Selector4 : Selector  InputPortWidth=9  IndexOptions=Index vector (dialog)  Indices=[1 5 9]  OutputSizes=1
  Selector5 : Selector  InputPortWidth=9  IndexOptions=Index vector (dialog)  Indices=[2 3 4 6 7 8]  OutputSizes=1
  wires:
  w_R_RFoot_des/1 -> Permute Dimensions1/1
  omega_Rot_task/1 -> Rot_task omega/1
  omega_RFoot/1 -> RFoot omega/1
  omega_LFoot/1 -> LFoot omega/1
  omegaDot_LFoot/1 -> LFoot omegaDot/1
  omegaDot_RFoot/1 -> RFoot omegaDot/1
  omegaDot_Root/1 -> Rot_task omegaDot/1
  Permute Dimensions2/1 -> Product2/2
  Permute Dimensions1/1 -> Product1/2
  Permute Dimensions3/1 -> Product/2
  Product2/1 -> Reshape1/1
  Product1/1 -> Reshape2/1
  Product/1 -> Reshape/1
  w_R_Rot_task/1 -> Product/1
  w_R_RFoot/1 -> Product1/1
  w_R_LFoot/1 -> Product2/1
  Reshape1/1 -> Selector/1, Selector1/1
  Reshape2/1 -> Selector2/1, Selector3/1
  Reshape/1 -> Selector4/1, Selector5/1
  Selector1/1 -> Rotation Error LFoot/2
  Selector/1 -> Rotation Error LFoot/1
  Selector2/1 -> Rotation Error RFoot/1
  Selector3/1 -> Rotation Error RFoot/2
  Selector4/1 -> Rotation Error Rot_task/1
  Selector5/1 -> Rotation Error Rot_task/2
  w_R_Rot_task_des/1 -> Permute Dimensions3/1
  w_R_LFoot_des/1 -> Permute Dimensions2/1

== system positionWalking_legacy/Robot State and References/State Machine/Select Current State and References/task position and orientation ==
  s : Inport
  w_H_b : Inport  Port=2
  CoM : WBToolboxLibrary/wholeBodyModel/Kinematics/Forward Kinematics  frameName=Frames.COM  robotName=WBT_robotName  localName=WBT_modelName  wbiFile=WBT_wbiFilename  wbiList=WBT_wbiList
  LFoot : WBToolboxLibrary/wholeBodyModel/Kinematics/Forward Kinematics  frameName=Frames.LEFT_FOOT  robotName=WBT_robotName  localName=WBT_modelName  wbiFile=WBT_wbiFilename  wbiList=WBT_wbiList
  RFoot : WBToolboxLibrary/wholeBodyModel/Kinematics/Forward Kinematics  frameName=Frames.RIGHT_FOOT  robotName=WBT_robotName  localName=WBT_modelName  wbiFile=WBT_wbiFilename  wbiList=WBT_wbiList
  Root : WBToolboxLibrary/wholeBodyModel/Kinematics/Forward Kinematics  frameName=Frames.ROT_TASK_LINK  robotName=WBT_robotName  localName=WBT_modelName  wbiFile=WBT_wbiFilename  wbiList=WBT_wbiList
  w_H_CoM : Outport
  w_H_l_sole : Outport  Port=2
  w_H_r_sole : Outport  Port=3
  w_H_rot_task : Outport  Port=4
  wires:
  s/1 -> Root/2, RFoot/2, LFoot/2, CoM/2
  w_H_b/1 -> Root/1, CoM/1, LFoot/1, RFoot/1
  CoM/1 -> w_H_CoM/1
  LFoot/1 -> w_H_l_sole/1
  RFoot/1 -> w_H_r_sole/1
  Root/1 -> w_H_rot_task/1

== system positionWalking_legacy/Robot State and References/State Machine/World to fixed link transform/w_H_b with left foot fixed ==
  s : Inport
  inertial : Inport  Port=2
  w_H_fixedLink : Inport  Port=3
  Constant6 : Constant  Value=eye(4)
  Head state : WBToolboxLibrary/Utilities/Yarp Read  portName=Ports.NECK_POS  signalSize=6  blocking=off  timestamp=off  autoconnect=on  errorOnConnection=off
  Inv\* : Product  Inputs=/*  Multiplication=Matrix(*)
  "Inv\\*  " : Product  Inputs=/*  Multiplication=Matrix(*)
  Switch6 : Switch  Criteria=u2 > Threshold
  USE_IMU4EST_BASE : Constant  Value=Config.USE_IMU4EST_BASE
  fromImuToHomogeousTransformFCN : MATLAB Function  TreatAsAtomicUnit=on
      settings: PermitHierarchicalResolution=ParametersOnly
  holder 1 : WBToolboxLibrary/Utilities/holder 
  holder 2 : WBToolboxLibrary/Utilities/holder 
  imu : WBToolboxLibrary/wholeBodyModel/Kinematics/Forward Kinematics  frameName=Frames.IMU  robotName=WBT_robotName  localName=WBT_modelName  wbiFile=WBT_wbiFilename  wbiList=WBT_wbiList
  neck transform : Subsystem
  root_link : WBToolboxLibrary/wholeBodyModel/Kinematics/Forward Kinematics  frameName=Frames.BASE_LINK  robotName=WBT_robotName  localName=WBT_modelName  wbiFile=WBT_wbiFilename  wbiList=WBT_wbiList
  w_H_b : Outport
  wires:
  Switch6/1 -> w_H_b/1
  "Inv\\*  "/1 -> Switch6/3, fromImuToHomogeousTransformFCN/3(link_H_base)  "link_H_root"
  USE_IMU4EST_BASE/1 -> Switch6/2
  Inv\*/1 -> holder 1/1, fromImuToHomogeousTransformFCN/1(imu_H_link)  "imu_H_link"
  holder 2/1 -> fromImuToHomogeousTransformFCN/4(inertial_0)
  imu/1 -> Inv\*/1
  holder 1/1 -> fromImuToHomogeousTransformFCN/2(imu_H_link_0)
  s/1 -> imu/2, root_link/2
  fromImuToHomogeousTransformFCN/1(w_H_b) -> Switch6/1
  Constant6/1 -> root_link/1, imu/1
  root_link/1 -> "Inv\\*  "/2
  inertial/1 -> holder 2/1, fromImuToHomogeousTransformFCN/5(inertial)
  Head state/1 -> neck transform/1(neck port)
  neck transform/1(neck position) -> fromImuToHomogeousTransformFCN/6(neck_pos)
  w_H_fixedLink/1 -> "Inv\\*  "/1, Inv\*/2

== system positionWalking_legacy/Robot State and References/State Machine/World to fixed link transform/w_H_b with right foot fixed ==
  s : Inport  PortDimensions=ROBOT_DOF
  inertial : Inport  Port=2  PortDimensions=12
  w_H_fixedLink : Inport  Port=3  PortDimensions=[4,4]
  Constant6 : Constant  Value=eye(4)
  Head state : WBToolboxLibrary/Utilities/Yarp Read  portName=Ports.NECK_POS  signalSize=6  blocking=off  timestamp=off  autoconnect=on  errorOnConnection=off
  Inv\* : Product  Inputs=/*  Multiplication=Matrix(*)
  "Inv\\*  " : Product  Inputs=/*  Multiplication=Matrix(*)
  Switch6 : Switch  Criteria=u2 > Threshold
  USE_IMU4EST_BASE : Constant  Value=Config.USE_IMU4EST_BASE
  fromImuToHomogeousTransformFCN : MATLAB Function  TreatAsAtomicUnit=on
      settings: PermitHierarchicalResolution=ParametersOnly
  holder 1 : WBToolboxLibrary/Utilities/holder 
  holder 2 : WBToolboxLibrary/Utilities/holder 
  imu : WBToolboxLibrary/wholeBodyModel/Kinematics/Forward Kinematics  frameName=Frames.IMU  robotName=WBT_robotName  localName=WBT_modelName  wbiFile=WBT_wbiFilename  wbiList=WBT_wbiList
  neck transform : Subsystem
  root_link : WBToolboxLibrary/wholeBodyModel/Kinematics/Forward Kinematics  frameName=Frames.BASE_LINK  robotName=WBT_robotName  localName=WBT_modelName  wbiFile=WBT_wbiFilename  wbiList=WBT_wbiList
  w_H_b : Outport
  wires:
  Switch6/1 -> w_H_b/1
  "Inv\\*  "/1 -> Switch6/3, fromImuToHomogeousTransformFCN/3(link_H_base)  "link_H_root"
  USE_IMU4EST_BASE/1 -> Switch6/2
  Inv\*/1 -> holder 1/1, fromImuToHomogeousTransformFCN/1(imu_H_link)  "imu_H_link"
  holder 2/1 -> fromImuToHomogeousTransformFCN/4(inertial_0)
  imu/1 -> Inv\*/1
  holder 1/1 -> fromImuToHomogeousTransformFCN/2(imu_H_link_0)
  s/1 -> imu/2, root_link/2
  fromImuToHomogeousTransformFCN/1(w_H_b) -> Switch6/1
  Constant6/1 -> root_link/1, imu/1
  root_link/1 -> "Inv\\*  "/2
  inertial/1 -> holder 2/1, fromImuToHomogeousTransformFCN/5(inertial)
  Head state/1 -> neck transform/1(neck port)
  neck transform/1(neck position) -> fromImuToHomogeousTransformFCN/6(neck_pos)
  w_H_fixedLink/1 -> "Inv\\*  "/1, Inv\*/2

== system positionWalking_legacy/Robot State and References/State Machine/compute state velocity/Feet Jacobians ==
  s : Inport
  w_H_b : Inport  Port=2
  Jacobian LFoot : WBToolboxLibrary/wholeBodyModel/Jacobians/Jacobian  frameName=Frames.LEFT_FOOT  robotName=WBT_robotName  localName=WBT_modelName  wbiFile=WBT_wbiFilename  wbiList=WBT_wbiList
  Jacobian RFoot : WBToolboxLibrary/wholeBodyModel/Jacobians/Jacobian  frameName=Frames.RIGHT_FOOT  robotName=WBT_robotName  localName=WBT_modelName  wbiFile=WBT_wbiFilename  wbiList=WBT_wbiList
  J_LFoot : Outport
  J_RFoot : Outport  Port=2
  wires:
  Jacobian LFoot/1 -> J_LFoot/1
  Jacobian RFoot/1 -> J_RFoot/1
  w_H_b/1 -> Jacobian RFoot/1, Jacobian LFoot/1
  s/1 -> Jacobian LFoot/2, Jacobian RFoot/2

== system positionWalking_legacy/Robot State and References/State Machine/World to fixed link transform/w_H_b with left foot fixed/neck transform ==
  neck port : Inport
  Constant : Constant  Value=zeros(3,1)
  Gain : Gain  Gain=pi/180
  Selector1 : Selector  InputPortWidth=6  IndexOptions=Index vector (dialog)  Indices=[1:3]  OutputSizes=1
  Switch : Switch  Criteria=u2 > Threshold
  USE_IMU4EST_BASE1 : Constant  Value=Config.CORRECT_IMU_WITH_NECK_POS
  neck position : Outport
  wires:
  neck port/1 -> Gain/1
  USE_IMU4EST_BASE1/1 -> Switch/2
  Switch/1 -> neck position/1
  Gain/1 -> Selector1/1
  Constant/1 -> Switch/3
  Selector1/1 -> Switch/1  "neck pos"

== system positionWalking_legacy/Robot State and References/State Machine/World to fixed link transform/w_H_b with right foot fixed/neck transform ==
  neck port : Inport
  Constant : Constant  Value=zeros(3,1)
  Gain : Gain  Gain=pi/180
  Selector1 : Selector  InputPortWidth=6  IndexOptions=Index vector (dialog)  Indices=[1:3]  OutputSizes=1
  Switch : Switch  Criteria=u2 > Threshold
  USE_IMU4EST_BASE1 : Constant  Value=Config.CORRECT_IMU_WITH_NECK_POS
  neck position : Outport
  wires:
  neck port/1 -> Gain/1
  USE_IMU4EST_BASE1/1 -> Switch/2
  Switch/1 -> neck position/1
  Gain/1 -> Selector1/1
  Constant/1 -> Switch/3
  Selector1/1 -> Switch/1  "neck pos"

== matlab function Dynamics and Kinematics/Inverse Kinematics/QP-Based Inverse Kinematics/Compute QP Hessian, gradient and constraints  ==
  data: s input double; nu input double; s_sDot_sDDot_ref input double; Hessian output double; impedances input double; dampings input double; J input double; JDot_nu input double; acc_task_star input double; gradient output double; ConstraintMatrix output double; biasVectorConstraint output double
function [Hessian, gradient, ConstraintMatrix, biasVectorConstraint] = ...
             computeQPHessianAndConstraintsFCN(s, nu, s_sDot_sDDot_ref, impedances, dampings, J, JDot_nu, acc_task_star)
    
    [Hessian, gradient, ConstraintMatrix, biasVectorConstraint] = ...
        computeQPHessianAndConstraints(s, nu, s_sDot_sDDot_ref, impedances, dampings, J, JDot_nu, acc_task_star);
end

== matlab function Dynamics and Kinematics/Initial Conditions/compute state velocity/Compute Base Velocity ==
  data: J_LeftFoot input double; J_RightFoot input double; feetInContact input double; nu_b output double; sDot input double; Sat parameter double
function nu_b = computeBaseVelocityFCN(J_LeftFoot,J_RightFoot, feetInContact, sDot, Sat)

    nu_b = computeBaseVelocity(J_LeftFoot,J_RightFoot, feetInContact, sDot, Sat);
end
